simulink model "course project"  (R2023b)
settings: Solver=VariableStepAuto  StartTime=0.0  StopTime=2  RelTol=1e-3
libraries: simulink x1
(part 2 of 2)

== system course project/Register12/JCK-Trigger2 ==
  Set J : Inport
  Control C : Inport  Port=2
  Reset K : Inport  Port=3
  Logical Operator1 : Logic  Operator=NAND  Inputs=3  AllPortsSameDT=off  OutDataTypeStr=boolean
  Logical Operator2 : Logic  Operator=NAND  AllPortsSameDT=off  OutDataTypeStr=boolean
  Logical Operator3 : Logic  Operator=NAND  AllPortsSameDT=off  OutDataTypeStr=boolean
  Logical Operator5 : Logic  Operator=NAND  Inputs=3  AllPortsSameDT=off  OutDataTypeStr=boolean
  Memory : Memory
  Non-Inverted : Outport
  wires:
  Memory/1 -> Logical Operator5/2, Logical Operator3/1  "Feedback"
  Logical Operator1/1 -> Logical Operator2/1  "R"
  Logical Operator2/1 -> Non-Inverted/1, Memory/1
  Logical Operator3/1 -> Logical Operator1/2, Logical Operator2/2  "Feedback"
  Logical Operator5/1 -> Logical Operator3/2
  Set J/1 -> Logical Operator1/1
  Reset K/1 -> Logical Operator5/1
  Control C/1 -> Logical Operator5/3, Logical Operator1/3

== system course project/Register12/JCK-Trigger3 ==
  Set J : Inport
  Control C : Inport  Port=2
  Reset K : Inport  Port=3
  Logical Operator1 : Logic  Operator=NAND  Inputs=3  AllPortsSameDT=off  OutDataTypeStr=boolean
  Logical Operator2 : Logic  Operator=NAND  AllPortsSameDT=off  OutDataTypeStr=boolean
  Logical Operator3 : Logic  Operator=NAND  AllPortsSameDT=off  OutDataTypeStr=boolean
  Logical Operator5 : Logic  Operator=NAND  Inputs=3  AllPortsSameDT=off  OutDataTypeStr=boolean
  Memory : Memory
  Non-Inverted : Outport
  wires:
  Memory/1 -> Logical Operator5/2, Logical Operator3/1  "Feedback"
  Logical Operator1/1 -> Logical Operator2/1  "R"
  Logical Operator2/1 -> Non-Inverted/1, Memory/1
  Logical Operator3/1 -> Logical Operator1/2, Logical Operator2/2  "Feedback"
  Logical Operator5/1 -> Logical Operator3/2
  Set J/1 -> Logical Operator1/1
  Reset K/1 -> Logical Operator5/1
  Control C/1 -> Logical Operator5/3, Logical Operator1/3

== system course project/Register13/JCK-Trigger ==
  Set J : Inport
  Control C : Inport  Port=2
  Reset K : Inport  Port=3
  Logical Operator1 : Logic  Operator=NAND  Inputs=3  AllPortsSameDT=off  OutDataTypeStr=boolean
  Logical Operator2 : Logic  Operator=NAND  AllPortsSameDT=off  OutDataTypeStr=boolean
  Logical Operator3 : Logic  Operator=NAND  AllPortsSameDT=off  OutDataTypeStr=boolean
  Logical Operator5 : Logic  Operator=NAND  Inputs=3  AllPortsSameDT=off  OutDataTypeStr=boolean
  Memory : Memory
  Non-Inverted : Outport
  wires:
  Memory/1 -> Logical Operator5/2, Logical Operator3/1  "Feedback"
  Logical Operator1/1 -> Logical Operator2/1  "R"
  Logical Operator2/1 -> Non-Inverted/1, Memory/1
  Logical Operator3/1 -> Logical Operator1/2, Logical Operator2/2  "Feedback"
  Logical Operator5/1 -> Logical Operator3/2
  Set J/1 -> Logical Operator1/1
  Reset K/1 -> Logical Operator5/1
  Control C/1 -> Logical Operator5/3, Logical Operator1/3

== system course project/Register13/JCK-Trigger1 ==
  Set J : Inport
  Control C : Inport  Port=2
  Reset K : Inport  Port=3
  Logical Operator1 : Logic  Operator=NAND  Inputs=3  AllPortsSameDT=off  OutDataTypeStr=boolean
  Logical Operator2 : Logic  Operator=NAND  AllPortsSameDT=off  OutDataTypeStr=boolean
  Logical Operator3 : Logic  Operator=NAND  AllPortsSameDT=off  OutDataTypeStr=boolean
  Logical Operator5 : Logic  Operator=NAND  Inputs=3  AllPortsSameDT=off  OutDataTypeStr=boolean
  Memory : Memory
  Non-Inverted : Outport
  wires:
  Memory/1 -> Logical Operator5/2, Logical Operator3/1  "Feedback"
  Logical Operator1/1 -> Logical Operator2/1  "R"
  Logical Operator2/1 -> Non-Inverted/1, Memory/1
  Logical Operator3/1 -> Logical Operator1/2, Logical Operator2/2  "Feedback"
  Logical Operator5/1 -> Logical Operator3/2
  Set J/1 -> Logical Operator1/1
  Reset K/1 -> Logical Operator5/1
  Control C/1 -> Logical Operator5/3, Logical Operator1/3

== system course project/Register13/JCK-Trigger2 ==
  Set J : Inport
  Control C : Inport  Port=2
  Reset K : Inport  Port=3
  Logical Operator1 : Logic  Operator=NAND  Inputs=3  AllPortsSameDT=off  OutDataTypeStr=boolean
  Logical Operator2 : Logic  Operator=NAND  AllPortsSameDT=off  OutDataTypeStr=boolean
  Logical Operator3 : Logic  Operator=NAND  AllPortsSameDT=off  OutDataTypeStr=boolean
  Logical Operator5 : Logic  Operator=NAND  Inputs=3  AllPortsSameDT=off  OutDataTypeStr=boolean
  Memory : Memory
  Non-Inverted : Outport
  wires:
  Memory/1 -> Logical Operator5/2, Logical Operator3/1  "Feedback"
  Logical Operator1/1 -> Logical Operator2/1  "R"
  Logical Operator2/1 -> Non-Inverted/1, Memory/1
  Logical Operator3/1 -> Logical Operator1/2, Logical Operator2/2  "Feedback"
  Logical Operator5/1 -> Logical Operator3/2
  Set J/1 -> Logical Operator1/1
  Reset K/1 -> Logical Operator5/1
  Control C/1 -> Logical Operator5/3, Logical Operator1/3

== system course project/Register13/JCK-Trigger3 ==
  Set J : Inport
  Control C : Inport  Port=2
  Reset K : Inport  Port=3
  Logical Operator1 : Logic  Operator=NAND  Inputs=3  AllPortsSameDT=off  OutDataTypeStr=boolean
  Logical Operator2 : Logic  Operator=NAND  AllPortsSameDT=off  OutDataTypeStr=boolean
  Logical Operator3 : Logic  Operator=NAND  AllPortsSameDT=off  OutDataTypeStr=boolean
  Logical Operator5 : Logic  Operator=NAND  Inputs=3  AllPortsSameDT=off  OutDataTypeStr=boolean
  Memory : Memory
  Non-Inverted : Outport
  wires:
  Memory/1 -> Logical Operator5/2, Logical Operator3/1  "Feedback"
  Logical Operator1/1 -> Logical Operator2/1  "R"
  Logical Operator2/1 -> Non-Inverted/1, Memory/1
  Logical Operator3/1 -> Logical Operator1/2, Logical Operator2/2  "Feedback"
  Logical Operator5/1 -> Logical Operator3/2
  Set J/1 -> Logical Operator1/1
  Reset K/1 -> Logical Operator5/1
  Control C/1 -> Logical Operator5/3, Logical Operator1/3

== system course project/Register14/JCK-Trigger ==
  Set J : Inport
  Control C : Inport  Port=2
  Reset K : Inport  Port=3
  Logical Operator1 : Logic  Operator=NAND  Inputs=3  AllPortsSameDT=off  OutDataTypeStr=boolean
  Logical Operator2 : Logic  Operator=NAND  AllPortsSameDT=off  OutDataTypeStr=boolean
  Logical Operator3 : Logic  Operator=NAND  AllPortsSameDT=off  OutDataTypeStr=boolean
  Logical Operator5 : Logic  Operator=NAND  Inputs=3  AllPortsSameDT=off  OutDataTypeStr=boolean
  Memory : Memory
  Non-Inverted : Outport
  wires:
  Memory/1 -> Logical Operator5/2, Logical Operator3/1  "Feedback"
  Logical Operator1/1 -> Logical Operator2/1  "R"
  Logical Operator2/1 -> Non-Inverted/1, Memory/1
  Logical Operator3/1 -> Logical Operator1/2, Logical Operator2/2  "Feedback"
  Logical Operator5/1 -> Logical Operator3/2
  Set J/1 -> Logical Operator1/1
  Reset K/1 -> Logical Operator5/1
  Control C/1 -> Logical Operator5/3, Logical Operator1/3

== system course project/Register14/JCK-Trigger1 ==
  Set J : Inport
  Control C : Inport  Port=2
  Reset K : Inport  Port=3
  Logical Operator1 : Logic  Operator=NAND  Inputs=3  AllPortsSameDT=off  OutDataTypeStr=boolean
  Logical Operator2 : Logic  Operator=NAND  AllPortsSameDT=off  OutDataTypeStr=boolean
  Logical Operator3 : Logic  Operator=NAND  AllPortsSameDT=off  OutDataTypeStr=boolean
  Logical Operator5 : Logic  Operator=NAND  Inputs=3  AllPortsSameDT=off  OutDataTypeStr=boolean
  Memory : Memory
  Non-Inverted : Outport
  wires:
  Memory/1 -> Logical Operator5/2, Logical Operator3/1  "Feedback"
  Logical Operator1/1 -> Logical Operator2/1  "R"
  Logical Operator2/1 -> Non-Inverted/1, Memory/1
  Logical Operator3/1 -> Logical Operator1/2, Logical Operator2/2  "Feedback"
  Logical Operator5/1 -> Logical Operator3/2
  Set J/1 -> Logical Operator1/1
  Reset K/1 -> Logical Operator5/1
  Control C/1 -> Logical Operator5/3, Logical Operator1/3

== system course project/Register14/JCK-Trigger2 ==
  Set J : Inport
  Control C : Inport  Port=2
  Reset K : Inport  Port=3
  Logical Operator1 : Logic  Operator=NAND  Inputs=3  AllPortsSameDT=off  OutDataTypeStr=boolean
  Logical Operator2 : Logic  Operator=NAND  AllPortsSameDT=off  OutDataTypeStr=boolean
  Logical Operator3 : Logic  Operator=NAND  AllPortsSameDT=off  OutDataTypeStr=boolean
  Logical Operator5 : Logic  Operator=NAND  Inputs=3  AllPortsSameDT=off  OutDataTypeStr=boolean
  Memory : Memory
  Non-Inverted : Outport
  wires:
  Memory/1 -> Logical Operator5/2, Logical Operator3/1  "Feedback"
  Logical Operator1/1 -> Logical Operator2/1  "R"
  Logical Operator2/1 -> Non-Inverted/1, Memory/1
  Logical Operator3/1 -> Logical Operator1/2, Logical Operator2/2  "Feedback"
  Logical Operator5/1 -> Logical Operator3/2
  Set J/1 -> Logical Operator1/1
  Reset K/1 -> Logical Operator5/1
  Control C/1 -> Logical Operator5/3, Logical Operator1/3

== system course project/Register14/JCK-Trigger3 ==
  Set J : Inport
  Control C : Inport  Port=2
  Reset K : Inport  Port=3
  Logical Operator1 : Logic  Operator=NAND  Inputs=3  AllPortsSameDT=off  OutDataTypeStr=boolean
  Logical Operator2 : Logic  Operator=NAND  AllPortsSameDT=off  OutDataTypeStr=boolean
  Logical Operator3 : Logic  Operator=NAND  AllPortsSameDT=off  OutDataTypeStr=boolean
  Logical Operator5 : Logic  Operator=NAND  Inputs=3  AllPortsSameDT=off  OutDataTypeStr=boolean
  Memory : Memory
  Non-Inverted : Outport
  wires:
  Memory/1 -> Logical Operator5/2, Logical Operator3/1  "Feedback"
  Logical Operator1/1 -> Logical Operator2/1  "R"
  Logical Operator2/1 -> Non-Inverted/1, Memory/1
  Logical Operator3/1 -> Logical Operator1/2, Logical Operator2/2  "Feedback"
  Logical Operator5/1 -> Logical Operator3/2
  Set J/1 -> Logical Operator1/1
  Reset K/1 -> Logical Operator5/1
  Control C/1 -> Logical Operator5/3, Logical Operator1/3

== system course project/Register15/JCK-Trigger ==
  Set J : Inport
  Control C : Inport  Port=2
  Reset K : Inport  Port=3
  Logical Operator1 : Logic  Operator=NAND  Inputs=3  AllPortsSameDT=off  OutDataTypeStr=boolean
  Logical Operator2 : Logic  Operator=NAND  AllPortsSameDT=off  OutDataTypeStr=boolean
  Logical Operator3 : Logic  Operator=NAND  AllPortsSameDT=off  OutDataTypeStr=boolean
  Logical Operator5 : Logic  Operator=NAND  Inputs=3  AllPortsSameDT=off  OutDataTypeStr=boolean
  Memory : Memory
  Non-Inverted : Outport
  wires:
  Memory/1 -> Logical Operator5/2, Logical Operator3/1  "Feedback"
  Logical Operator1/1 -> Logical Operator2/1  "R"
  Logical Operator2/1 -> Non-Inverted/1, Memory/1
  Logical Operator3/1 -> Logical Operator1/2, Logical Operator2/2  "Feedback"
  Logical Operator5/1 -> Logical Operator3/2
  Set J/1 -> Logical Operator1/1
  Reset K/1 -> Logical Operator5/1
  Control C/1 -> Logical Operator5/3, Logical Operator1/3

== system course project/Register15/JCK-Trigger1 ==
  Set J : Inport
  Control C : Inport  Port=2
  Reset K : Inport  Port=3
  Logical Operator1 : Logic  Operator=NAND  Inputs=3  AllPortsSameDT=off  OutDataTypeStr=boolean
  Logical Operator2 : Logic  Operator=NAND  AllPortsSameDT=off  OutDataTypeStr=boolean
  Logical Operator3 : Logic  Operator=NAND  AllPortsSameDT=off  OutDataTypeStr=boolean
  Logical Operator5 : Logic  Operator=NAND  Inputs=3  AllPortsSameDT=off  OutDataTypeStr=boolean
  Memory : Memory
  Non-Inverted : Outport
  wires:
  Memory/1 -> Logical Operator5/2, Logical Operator3/1  "Feedback"
  Logical Operator1/1 -> Logical Operator2/1  "R"
  Logical Operator2/1 -> Non-Inverted/1, Memory/1
  Logical Operator3/1 -> Logical Operator1/2, Logical Operator2/2  "Feedback"
  Logical Operator5/1 -> Logical Operator3/2
  Set J/1 -> Logical Operator1/1
  Reset K/1 -> Logical Operator5/1
  Control C/1 -> Logical Operator5/3, Logical Operator1/3

== system course project/Register15/JCK-Trigger2 ==
  Set J : Inport
  Control C : Inport  Port=2
  Reset K : Inport  Port=3
  Logical Operator1 : Logic  Operator=NAND  Inputs=3  AllPortsSameDT=off  OutDataTypeStr=boolean
  Logical Operator2 : Logic  Operator=NAND  AllPortsSameDT=off  OutDataTypeStr=boolean
  Logical Operator3 : Logic  Operator=NAND  AllPortsSameDT=off  OutDataTypeStr=boolean
  Logical Operator5 : Logic  Operator=NAND  Inputs=3  AllPortsSameDT=off  OutDataTypeStr=boolean
  Memory : Memory
  Non-Inverted : Outport
  wires:
  Memory/1 -> Logical Operator5/2, Logical Operator3/1  "Feedback"
  Logical Operator1/1 -> Logical Operator2/1  "R"
  Logical Operator2/1 -> Non-Inverted/1, Memory/1
  Logical Operator3/1 -> Logical Operator1/2, Logical Operator2/2  "Feedback"
  Logical Operator5/1 -> Logical Operator3/2
  Set J/1 -> Logical Operator1/1
  Reset K/1 -> Logical Operator5/1
  Control C/1 -> Logical Operator5/3, Logical Operator1/3

== system course project/Register15/JCK-Trigger3 ==
  Set J : Inport
  Control C : Inport  Port=2
  Reset K : Inport  Port=3
  Logical Operator1 : Logic  Operator=NAND  Inputs=3  AllPortsSameDT=off  OutDataTypeStr=boolean
  Logical Operator2 : Logic  Operator=NAND  AllPortsSameDT=off  OutDataTypeStr=boolean
  Logical Operator3 : Logic  Operator=NAND  AllPortsSameDT=off  OutDataTypeStr=boolean
  Logical Operator5 : Logic  Operator=NAND  Inputs=3  AllPortsSameDT=off  OutDataTypeStr=boolean
  Memory : Memory
  Non-Inverted : Outport
  wires:
  Memory/1 -> Logical Operator5/2, Logical Operator3/1  "Feedback"
  Logical Operator1/1 -> Logical Operator2/1  "R"
  Logical Operator2/1 -> Non-Inverted/1, Memory/1
  Logical Operator3/1 -> Logical Operator1/2, Logical Operator2/2  "Feedback"
  Logical Operator5/1 -> Logical Operator3/2
  Set J/1 -> Logical Operator1/1
  Reset K/1 -> Logical Operator5/1
  Control C/1 -> Logical Operator5/3, Logical Operator1/3

== system course project/Register2/JCK-Trigger ==
  Set J : Inport
  Control C : Inport  Port=2
  Reset K : Inport  Port=3
  Logical Operator1 : Logic  Operator=NAND  Inputs=3  AllPortsSameDT=off  OutDataTypeStr=boolean
  Logical Operator2 : Logic  Operator=NAND  AllPortsSameDT=off  OutDataTypeStr=boolean
  Logical Operator3 : Logic  Operator=NAND  AllPortsSameDT=off  OutDataTypeStr=boolean
  Logical Operator5 : Logic  Operator=NAND  Inputs=3  AllPortsSameDT=off  OutDataTypeStr=boolean
  Memory : Memory
  Non-Inverted : Outport
  wires:
  Memory/1 -> Logical Operator5/2, Logical Operator3/1  "Feedback"
  Logical Operator1/1 -> Logical Operator2/1  "R"
  Logical Operator2/1 -> Non-Inverted/1, Memory/1
  Logical Operator3/1 -> Logical Operator1/2, Logical Operator2/2  "Feedback"
  Logical Operator5/1 -> Logical Operator3/2
  Set J/1 -> Logical Operator1/1
  Reset K/1 -> Logical Operator5/1
  Control C/1 -> Logical Operator5/3, Logical Operator1/3

== system course project/Register2/JCK-Trigger1 ==
  Set J : Inport
  Control C : Inport  Port=2
  Reset K : Inport  Port=3
  Logical Operator1 : Logic  Operator=NAND  Inputs=3  AllPortsSameDT=off  OutDataTypeStr=boolean
  Logical Operator2 : Logic  Operator=NAND  AllPortsSameDT=off  OutDataTypeStr=boolean
  Logical Operator3 : Logic  Operator=NAND  AllPortsSameDT=off  OutDataTypeStr=boolean
  Logical Operator5 : Logic  Operator=NAND  Inputs=3  AllPortsSameDT=off  OutDataTypeStr=boolean
  Memory : Memory
  Non-Inverted : Outport
  wires:
  Memory/1 -> Logical Operator5/2, Logical Operator3/1  "Feedback"
  Logical Operator1/1 -> Logical Operator2/1  "R"
  Logical Operator2/1 -> Non-Inverted/1, Memory/1
  Logical Operator3/1 -> Logical Operator1/2, Logical Operator2/2  "Feedback"
  Logical Operator5/1 -> Logical Operator3/2
  Set J/1 -> Logical Operator1/1
  Reset K/1 -> Logical Operator5/1
  Control C/1 -> Logical Operator5/3, Logical Operator1/3

== system course project/Register2/JCK-Trigger2 ==
  Set J : Inport
  Control C : Inport  Port=2
  Reset K : Inport  Port=3
  Logical Operator1 : Logic  Operator=NAND  Inputs=3  AllPortsSameDT=off  OutDataTypeStr=boolean
  Logical Operator2 : Logic  Operator=NAND  AllPortsSameDT=off  OutDataTypeStr=boolean
  Logical Operator3 : Logic  Operator=NAND  AllPortsSameDT=off  OutDataTypeStr=boolean
  Logical Operator5 : Logic  Operator=NAND  Inputs=3  AllPortsSameDT=off  OutDataTypeStr=boolean
  Memory : Memory
  Non-Inverted : Outport
  wires:
  Memory/1 -> Logical Operator5/2, Logical Operator3/1  "Feedback"
  Logical Operator1/1 -> Logical Operator2/1  "R"
  Logical Operator2/1 -> Non-Inverted/1, Memory/1
  Logical Operator3/1 -> Logical Operator1/2, Logical Operator2/2  "Feedback"
  Logical Operator5/1 -> Logical Operator3/2
  Set J/1 -> Logical Operator1/1
  Reset K/1 -> Logical Operator5/1
  Control C/1 -> Logical Operator5/3, Logical Operator1/3

== system course project/Register2/JCK-Trigger3 ==
  Set J : Inport
  Control C : Inport  Port=2
  Reset K : Inport  Port=3
  Logical Operator1 : Logic  Operator=NAND  Inputs=3  AllPortsSameDT=off  OutDataTypeStr=boolean
  Logical Operator2 : Logic  Operator=NAND  AllPortsSameDT=off  OutDataTypeStr=boolean
  Logical Operator3 : Logic  Operator=NAND  AllPortsSameDT=off  OutDataTypeStr=boolean
  Logical Operator5 : Logic  Operator=NAND  Inputs=3  AllPortsSameDT=off  OutDataTypeStr=boolean
  Memory : Memory
  Non-Inverted : Outport
  wires:
  Memory/1 -> Logical Operator5/2, Logical Operator3/1  "Feedback"
  Logical Operator1/1 -> Logical Operator2/1  "R"
  Logical Operator2/1 -> Non-Inverted/1, Memory/1
  Logical Operator3/1 -> Logical Operator1/2, Logical Operator2/2  "Feedback"
  Logical Operator5/1 -> Logical Operator3/2
  Set J/1 -> Logical Operator1/1
  Reset K/1 -> Logical Operator5/1
  Control C/1 -> Logical Operator5/3, Logical Operator1/3

== system course project/Register3/JCK-Trigger ==
  Set J : Inport
  Control C : Inport  Port=2
  Reset K : Inport  Port=3
  Logical Operator1 : Logic  Operator=NAND  Inputs=3  AllPortsSameDT=off  OutDataTypeStr=boolean
  Logical Operator2 : Logic  Operator=NAND  AllPortsSameDT=off  OutDataTypeStr=boolean
  Logical Operator3 : Logic  Operator=NAND  AllPortsSameDT=off  OutDataTypeStr=boolean
  Logical Operator5 : Logic  Operator=NAND  Inputs=3  AllPortsSameDT=off  OutDataTypeStr=boolean
  Memory : Memory
  Non-Inverted : Outport
  wires:
  Memory/1 -> Logical Operator5/2, Logical Operator3/1  "Feedback"
  Logical Operator1/1 -> Logical Operator2/1  "R"
  Logical Operator2/1 -> Non-Inverted/1, Memory/1
  Logical Operator3/1 -> Logical Operator1/2, Logical Operator2/2  "Feedback"
  Logical Operator5/1 -> Logical Operator3/2
  Set J/1 -> Logical Operator1/1
  Reset K/1 -> Logical Operator5/1
  Control C/1 -> Logical Operator5/3, Logical Operator1/3

== system course project/Register3/JCK-Trigger1 ==
  Set J : Inport
  Control C : Inport  Port=2
  Reset K : Inport  Port=3
  Logical Operator1 : Logic  Operator=NAND  Inputs=3  AllPortsSameDT=off  OutDataTypeStr=boolean
  Logical Operator2 : Logic  Operator=NAND  AllPortsSameDT=off  OutDataTypeStr=boolean
  Logical Operator3 : Logic  Operator=NAND  AllPortsSameDT=off  OutDataTypeStr=boolean
  Logical Operator5 : Logic  Operator=NAND  Inputs=3  AllPortsSameDT=off  OutDataTypeStr=boolean
  Memory : Memory
  Non-Inverted : Outport
  wires:
  Memory/1 -> Logical Operator5/2, Logical Operator3/1  "Feedback"
  Logical Operator1/1 -> Logical Operator2/1  "R"
  Logical Operator2/1 -> Non-Inverted/1, Memory/1
  Logical Operator3/1 -> Logical Operator1/2, Logical Operator2/2  "Feedback"
  Logical Operator5/1 -> Logical Operator3/2
  Set J/1 -> Logical Operator1/1
  Reset K/1 -> Logical Operator5/1
  Control C/1 -> Logical Operator5/3, Logical Operator1/3

== system course project/Register3/JCK-Trigger2 ==
  Set J : Inport
  Control C : Inport  Port=2
  Reset K : Inport  Port=3
  Logical Operator1 : Logic  Operator=NAND  Inputs=3  AllPortsSameDT=off  OutDataTypeStr=boolean
  Logical Operator2 : Logic  Operator=NAND  AllPortsSameDT=off  OutDataTypeStr=boolean
  Logical Operator3 : Logic  Operator=NAND  AllPortsSameDT=off  OutDataTypeStr=boolean
  Logical Operator5 : Logic  Operator=NAND  Inputs=3  AllPortsSameDT=off  OutDataTypeStr=boolean
  Memory : Memory
  Non-Inverted : Outport
  wires:
  Memory/1 -> Logical Operator5/2, Logical Operator3/1  "Feedback"
  Logical Operator1/1 -> Logical Operator2/1  "R"
  Logical Operator2/1 -> Non-Inverted/1, Memory/1
  Logical Operator3/1 -> Logical Operator1/2, Logical Operator2/2  "Feedback"
  Logical Operator5/1 -> Logical Operator3/2
  Set J/1 -> Logical Operator1/1
  Reset K/1 -> Logical Operator5/1
  Control C/1 -> Logical Operator5/3, Logical Operator1/3

== system course project/Register3/JCK-Trigger3 ==
  Set J : Inport
  Control C : Inport  Port=2
  Reset K : Inport  Port=3
  Logical Operator1 : Logic  Operator=NAND  Inputs=3  AllPortsSameDT=off  OutDataTypeStr=boolean
  Logical Operator2 : Logic  Operator=NAND  AllPortsSameDT=off  OutDataTypeStr=boolean
  Logical Operator3 : Logic  Operator=NAND  AllPortsSameDT=off  OutDataTypeStr=boolean
  Logical Operator5 : Logic  Operator=NAND  Inputs=3  AllPortsSameDT=off  OutDataTypeStr=boolean
  Memory : Memory
  Non-Inverted : Outport
  wires:
  Memory/1 -> Logical Operator5/2, Logical Operator3/1  "Feedback"
  Logical Operator1/1 -> Logical Operator2/1  "R"
  Logical Operator2/1 -> Non-Inverted/1, Memory/1
  Logical Operator3/1 -> Logical Operator1/2, Logical Operator2/2  "Feedback"
  Logical Operator5/1 -> Logical Operator3/2
  Set J/1 -> Logical Operator1/1
  Reset K/1 -> Logical Operator5/1
  Control C/1 -> Logical Operator5/3, Logical Operator1/3

== system course project/Register4/JCK-Trigger ==
  Set J : Inport
  Control C : Inport  Port=2
  Reset K : Inport  Port=3
  Logical Operator1 : Logic  Operator=NAND  Inputs=3  AllPortsSameDT=off  OutDataTypeStr=boolean
  Logical Operator2 : Logic  Operator=NAND  AllPortsSameDT=off  OutDataTypeStr=boolean
  Logical Operator3 : Logic  Operator=NAND  AllPortsSameDT=off  OutDataTypeStr=boolean
  Logical Operator5 : Logic  Operator=NAND  Inputs=3  AllPortsSameDT=off  OutDataTypeStr=boolean
  Memory : Memory
  Non-Inverted : Outport
  wires:
  Memory/1 -> Logical Operator5/2, Logical Operator3/1  "Feedback"
  Logical Operator1/1 -> Logical Operator2/1  "R"
  Logical Operator2/1 -> Non-Inverted/1, Memory/1
  Logical Operator3/1 -> Logical Operator1/2, Logical Operator2/2  "Feedback"
  Logical Operator5/1 -> Logical Operator3/2
  Set J/1 -> Logical Operator1/1
  Reset K/1 -> Logical Operator5/1
  Control C/1 -> Logical Operator5/3, Logical Operator1/3

== system course project/Register4/JCK-Trigger1 ==
  Set J : Inport
  Control C : Inport  Port=2
  Reset K : Inport  Port=3
  Logical Operator1 : Logic  Operator=NAND  Inputs=3  AllPortsSameDT=off  OutDataTypeStr=boolean
  Logical Operator2 : Logic  Operator=NAND  AllPortsSameDT=off  OutDataTypeStr=boolean
  Logical Operator3 : Logic  Operator=NAND  AllPortsSameDT=off  OutDataTypeStr=boolean
  Logical Operator5 : Logic  Operator=NAND  Inputs=3  AllPortsSameDT=off  OutDataTypeStr=boolean
  Memory : Memory
  Non-Inverted : Outport
  wires:
  Memory/1 -> Logical Operator5/2, Logical Operator3/1  "Feedback"
  Logical Operator1/1 -> Logical Operator2/1  "R"
  Logical Operator2/1 -> Non-Inverted/1, Memory/1
  Logical Operator3/1 -> Logical Operator1/2, Logical Operator2/2  "Feedback"
  Logical Operator5/1 -> Logical Operator3/2
  Set J/1 -> Logical Operator1/1
  Reset K/1 -> Logical Operator5/1
  Control C/1 -> Logical Operator5/3, Logical Operator1/3

== system course project/Register4/JCK-Trigger2 ==
  Set J : Inport
  Control C : Inport  Port=2
  Reset K : Inport  Port=3
  Logical Operator1 : Logic  Operator=NAND  Inputs=3  AllPortsSameDT=off  OutDataTypeStr=boolean
  Logical Operator2 : Logic  Operator=NAND  AllPortsSameDT=off  OutDataTypeStr=boolean
  Logical Operator3 : Logic  Operator=NAND  AllPortsSameDT=off  OutDataTypeStr=boolean
  Logical Operator5 : Logic  Operator=NAND  Inputs=3  AllPortsSameDT=off  OutDataTypeStr=boolean
  Memory : Memory
  Non-Inverted : Outport
  wires:
  Memory/1 -> Logical Operator5/2, Logical Operator3/1  "Feedback"
  Logical Operator1/1 -> Logical Operator2/1  "R"
  Logical Operator2/1 -> Non-Inverted/1, Memory/1
  Logical Operator3/1 -> Logical Operator1/2, Logical Operator2/2  "Feedback"
  Logical Operator5/1 -> Logical Operator3/2
  Set J/1 -> Logical Operator1/1
  Reset K/1 -> Logical Operator5/1
  Control C/1 -> Logical Operator5/3, Logical Operator1/3

== system course project/Register4/JCK-Trigger3 ==
  Set J : Inport
  Control C : Inport  Port=2
  Reset K : Inport  Port=3
  Logical Operator1 : Logic  Operator=NAND  Inputs=3  AllPortsSameDT=off  OutDataTypeStr=boolean
  Logical Operator2 : Logic  Operator=NAND  AllPortsSameDT=off  OutDataTypeStr=boolean
  Logical Operator3 : Logic  Operator=NAND  AllPortsSameDT=off  OutDataTypeStr=boolean
  Logical Operator5 : Logic  Operator=NAND  Inputs=3  AllPortsSameDT=off  OutDataTypeStr=boolean
  Memory : Memory
  Non-Inverted : Outport
  wires:
  Memory/1 -> Logical Operator5/2, Logical Operator3/1  "Feedback"
  Logical Operator1/1 -> Logical Operator2/1  "R"
  Logical Operator2/1 -> Non-Inverted/1, Memory/1
  Logical Operator3/1 -> Logical Operator1/2, Logical Operator2/2  "Feedback"
  Logical Operator5/1 -> Logical Operator3/2
  Set J/1 -> Logical Operator1/1
  Reset K/1 -> Logical Operator5/1
  Control C/1 -> Logical Operator5/3, Logical Operator1/3

== system course project/Register5/JCK-Trigger ==
  Set J : Inport
  Control C : Inport  Port=2
  Reset K : Inport  Port=3
  Logical Operator1 : Logic  Operator=NAND  Inputs=3  AllPortsSameDT=off  OutDataTypeStr=boolean
  Logical Operator2 : Logic  Operator=NAND  AllPortsSameDT=off  OutDataTypeStr=boolean
  Logical Operator3 : Logic  Operator=NAND  AllPortsSameDT=off  OutDataTypeStr=boolean
  Logical Operator5 : Logic  Operator=NAND  Inputs=3  AllPortsSameDT=off  OutDataTypeStr=boolean
  Memory : Memory
  Non-Inverted : Outport
  wires:
  Memory/1 -> Logical Operator5/2, Logical Operator3/1  "Feedback"
  Logical Operator1/1 -> Logical Operator2/1  "R"
  Logical Operator2/1 -> Non-Inverted/1, Memory/1
  Logical Operator3/1 -> Logical Operator1/2, Logical Operator2/2  "Feedback"
  Logical Operator5/1 -> Logical Operator3/2
  Set J/1 -> Logical Operator1/1
  Reset K/1 -> Logical Operator5/1
  Control C/1 -> Logical Operator5/3, Logical Operator1/3

== system course project/Register5/JCK-Trigger1 ==
  Set J : Inport
  Control C : Inport  Port=2
  Reset K : Inport  Port=3
  Logical Operator1 : Logic  Operator=NAND  Inputs=3  AllPortsSameDT=off  OutDataTypeStr=boolean
  Logical Operator2 : Logic  Operator=NAND  AllPortsSameDT=off  OutDataTypeStr=boolean
  Logical Operator3 : Logic  Operator=NAND  AllPortsSameDT=off  OutDataTypeStr=boolean
  Logical Operator5 : Logic  Operator=NAND  Inputs=3  AllPortsSameDT=off  OutDataTypeStr=boolean
  Memory : Memory
  Non-Inverted : Outport
  wires:
  Memory/1 -> Logical Operator5/2, Logical Operator3/1  "Feedback"
  Logical Operator1/1 -> Logical Operator2/1  "R"
  Logical Operator2/1 -> Non-Inverted/1, Memory/1
  Logical Operator3/1 -> Logical Operator1/2, Logical Operator2/2  "Feedback"
  Logical Operator5/1 -> Logical Operator3/2
  Set J/1 -> Logical Operator1/1
  Reset K/1 -> Logical Operator5/1
  Control C/1 -> Logical Operator5/3, Logical Operator1/3

== system course project/Register5/JCK-Trigger2 ==
  Set J : Inport
  Control C : Inport  Port=2
  Reset K : Inport  Port=3
  Logical Operator1 : Logic  Operator=NAND  Inputs=3  AllPortsSameDT=off  OutDataTypeStr=boolean
  Logical Operator2 : Logic  Operator=NAND  AllPortsSameDT=off  OutDataTypeStr=boolean
  Logical Operator3 : Logic  Operator=NAND  AllPortsSameDT=off  OutDataTypeStr=boolean
  Logical Operator5 : Logic  Operator=NAND  Inputs=3  AllPortsSameDT=off  OutDataTypeStr=boolean
  Memory : Memory
  Non-Inverted : Outport
  wires:
  Memory/1 -> Logical Operator5/2, Logical Operator3/1  "Feedback"
  Logical Operator1/1 -> Logical Operator2/1  "R"
  Logical Operator2/1 -> Non-Inverted/1, Memory/1
  Logical Operator3/1 -> Logical Operator1/2, Logical Operator2/2  "Feedback"
  Logical Operator5/1 -> Logical Operator3/2
  Set J/1 -> Logical Operator1/1
  Reset K/1 -> Logical Operator5/1
  Control C/1 -> Logical Operator5/3, Logical Operator1/3

== system course project/Register5/JCK-Trigger3 ==
  Set J : Inport
  Control C : Inport  Port=2
  Reset K : Inport  Port=3
  Logical Operator1 : Logic  Operator=NAND  Inputs=3  AllPortsSameDT=off  OutDataTypeStr=boolean
  Logical Operator2 : Logic  Operator=NAND  AllPortsSameDT=off  OutDataTypeStr=boolean
  Logical Operator3 : Logic  Operator=NAND  AllPortsSameDT=off  OutDataTypeStr=boolean
  Logical Operator5 : Logic  Operator=NAND  Inputs=3  AllPortsSameDT=off  OutDataTypeStr=boolean
  Memory : Memory
  Non-Inverted : Outport
  wires:
  Memory/1 -> Logical Operator5/2, Logical Operator3/1  "Feedback"
  Logical Operator1/1 -> Logical Operator2/1  "R"
  Logical Operator2/1 -> Non-Inverted/1, Memory/1
  Logical Operator3/1 -> Logical Operator1/2, Logical Operator2/2  "Feedback"
  Logical Operator5/1 -> Logical Operator3/2
  Set J/1 -> Logical Operator1/1
  Reset K/1 -> Logical Operator5/1
  Control C/1 -> Logical Operator5/3, Logical Operator1/3

== system course project/Register6/JCK-Trigger ==
  Set J : Inport
  Control C : Inport  Port=2
  Reset K : Inport  Port=3
  Logical Operator1 : Logic  Operator=NAND  Inputs=3  AllPortsSameDT=off  OutDataTypeStr=boolean
  Logical Operator2 : Logic  Operator=NAND  AllPortsSameDT=off  OutDataTypeStr=boolean
  Logical Operator3 : Logic  Operator=NAND  AllPortsSameDT=off  OutDataTypeStr=boolean
  Logical Operator5 : Logic  Operator=NAND  Inputs=3  AllPortsSameDT=off  OutDataTypeStr=boolean
  Memory : Memory
  Non-Inverted : Outport
  wires:
  Memory/1 -> Logical Operator5/2, Logical Operator3/1  "Feedback"
  Logical Operator1/1 -> Logical Operator2/1  "R"
  Logical Operator2/1 -> Non-Inverted/1, Memory/1
  Logical Operator3/1 -> Logical Operator1/2, Logical Operator2/2  "Feedback"
  Logical Operator5/1 -> Logical Operator3/2
  Set J/1 -> Logical Operator1/1
  Reset K/1 -> Logical Operator5/1
  Control C/1 -> Logical Operator5/3, Logical Operator1/3

== system course project/Register6/JCK-Trigger1 ==
  Set J : Inport
  Control C : Inport  Port=2
  Reset K : Inport  Port=3
  Logical Operator1 : Logic  Operator=NAND  Inputs=3  AllPortsSameDT=off  OutDataTypeStr=boolean
  Logical Operator2 : Logic  Operator=NAND  AllPortsSameDT=off  OutDataTypeStr=boolean
  Logical Operator3 : Logic  Operator=NAND  AllPortsSameDT=off  OutDataTypeStr=boolean
  Logical Operator5 : Logic  Operator=NAND  Inputs=3  AllPortsSameDT=off  OutDataTypeStr=boolean
  Memory : Memory
  Non-Inverted : Outport
  wires:
  Memory/1 -> Logical Operator5/2, Logical Operator3/1  "Feedback"
  Logical Operator1/1 -> Logical Operator2/1  "R"
  Logical Operator2/1 -> Non-Inverted/1, Memory/1
  Logical Operator3/1 -> Logical Operator1/2, Logical Operator2/2  "Feedback"
  Logical Operator5/1 -> Logical Operator3/2
  Set J/1 -> Logical Operator1/1
  Reset K/1 -> Logical Operator5/1
  Control C/1 -> Logical Operator5/3, Logical Operator1/3

== system course project/Register6/JCK-Trigger2 ==
  Set J : Inport
  Control C : Inport  Port=2
  Reset K : Inport  Port=3
  Logical Operator1 : Logic  Operator=NAND  Inputs=3  AllPortsSameDT=off  OutDataTypeStr=boolean
  Logical Operator2 : Logic  Operator=NAND  AllPortsSameDT=off  OutDataTypeStr=boolean
  Logical Operator3 : Logic  Operator=NAND  AllPortsSameDT=off  OutDataTypeStr=boolean
  Logical Operator5 : Logic  Operator=NAND  Inputs=3  AllPortsSameDT=off  OutDataTypeStr=boolean
  Memory : Memory
  Non-Inverted : Outport
  wires:
  Memory/1 -> Logical Operator5/2, Logical Operator3/1  "Feedback"
  Logical Operator1/1 -> Logical Operator2/1  "R"
  Logical Operator2/1 -> Non-Inverted/1, Memory/1
  Logical Operator3/1 -> Logical Operator1/2, Logical Operator2/2  "Feedback"
  Logical Operator5/1 -> Logical Operator3/2
  Set J/1 -> Logical Operator1/1
  Reset K/1 -> Logical Operator5/1
  Control C/1 -> Logical Operator5/3, Logical Operator1/3

== system course project/Register6/JCK-Trigger3 ==
  Set J : Inport
  Control C : Inport  Port=2
  Reset K : Inport  Port=3
  Logical Operator1 : Logic  Operator=NAND  Inputs=3  AllPortsSameDT=off  OutDataTypeStr=boolean
  Logical Operator2 : Logic  Operator=NAND  AllPortsSameDT=off  OutDataTypeStr=boolean
  Logical Operator3 : Logic  Operator=NAND  AllPortsSameDT=off  OutDataTypeStr=boolean
  Logical Operator5 : Logic  Operator=NAND  Inputs=3  AllPortsSameDT=off  OutDataTypeStr=boolean
  Memory : Memory
  Non-Inverted : Outport
  wires:
  Memory/1 -> Logical Operator5/2, Logical Operator3/1  "Feedback"
  Logical Operator1/1 -> Logical Operator2/1  "R"
  Logical Operator2/1 -> Non-Inverted/1, Memory/1
  Logical Operator3/1 -> Logical Operator1/2, Logical Operator2/2  "Feedback"
  Logical Operator5/1 -> Logical Operator3/2
  Set J/1 -> Logical Operator1/1
  Reset K/1 -> Logical Operator5/1
  Control C/1 -> Logical Operator5/3, Logical Operator1/3

== system course project/Register7/JCK-Trigger ==
  Set J : Inport
  Control C : Inport  Port=2
  Reset K : Inport  Port=3
  Logical Operator1 : Logic  Operator=NAND  Inputs=3  AllPortsSameDT=off  OutDataTypeStr=boolean
  Logical Operator2 : Logic  Operator=NAND  AllPortsSameDT=off  OutDataTypeStr=boolean
  Logical Operator3 : Logic  Operator=NAND  AllPortsSameDT=off  OutDataTypeStr=boolean
  Logical Operator5 : Logic  Operator=NAND  Inputs=3  AllPortsSameDT=off  OutDataTypeStr=boolean
  Memory : Memory
  Non-Inverted : Outport
  wires:
  Memory/1 -> Logical Operator5/2, Logical Operator3/1  "Feedback"
  Logical Operator1/1 -> Logical Operator2/1  "R"
  Logical Operator2/1 -> Non-Inverted/1, Memory/1
  Logical Operator3/1 -> Logical Operator1/2, Logical Operator2/2  "Feedback"
  Logical Operator5/1 -> Logical Operator3/2
  Set J/1 -> Logical Operator1/1
  Reset K/1 -> Logical Operator5/1
  Control C/1 -> Logical Operator5/3, Logical Operator1/3

== system course project/Register7/JCK-Trigger1 ==
  Set J : Inport
  Control C : Inport  Port=2
  Reset K : Inport  Port=3
  Logical Operator1 : Logic  Operator=NAND  Inputs=3  AllPortsSameDT=off  OutDataTypeStr=boolean
  Logical Operator2 : Logic  Operator=NAND  AllPortsSameDT=off  OutDataTypeStr=boolean
  Logical Operator3 : Logic  Operator=NAND  AllPortsSameDT=off  OutDataTypeStr=boolean
  Logical Operator5 : Logic  Operator=NAND  Inputs=3  AllPortsSameDT=off  OutDataTypeStr=boolean
  Memory : Memory
  Non-Inverted : Outport
  wires:
  Memory/1 -> Logical Operator5/2, Logical Operator3/1  "Feedback"
  Logical Operator1/1 -> Logical Operator2/1  "R"
  Logical Operator2/1 -> Non-Inverted/1, Memory/1
  Logical Operator3/1 -> Logical Operator1/2, Logical Operator2/2  "Feedback"
  Logical Operator5/1 -> Logical Operator3/2
  Set J/1 -> Logical Operator1/1
  Reset K/1 -> Logical Operator5/1
  Control C/1 -> Logical Operator5/3, Logical Operator1/3

== system course project/Register7/JCK-Trigger2 ==
  Set J : Inport
  Control C : Inport  Port=2
  Reset K : Inport  Port=3
  Logical Operator1 : Logic  Operator=NAND  Inputs=3  AllPortsSameDT=off  OutDataTypeStr=boolean
  Logical Operator2 : Logic  Operator=NAND  AllPortsSameDT=off  OutDataTypeStr=boolean
  Logical Operator3 : Logic  Operator=NAND  AllPortsSameDT=off  OutDataTypeStr=boolean
  Logical Operator5 : Logic  Operator=NAND  Inputs=3  AllPortsSameDT=off  OutDataTypeStr=boolean
  Memory : Memory
  Non-Inverted : Outport
  wires:
  Memory/1 -> Logical Operator5/2, Logical Operator3/1  "Feedback"
  Logical Operator1/1 -> Logical Operator2/1  "R"
  Logical Operator2/1 -> Non-Inverted/1, Memory/1
  Logical Operator3/1 -> Logical Operator1/2, Logical Operator2/2  "Feedback"
  Logical Operator5/1 -> Logical Operator3/2
  Set J/1 -> Logical Operator1/1
  Reset K/1 -> Logical Operator5/1
  Control C/1 -> Logical Operator5/3, Logical Operator1/3

== system course project/Register7/JCK-Trigger3 ==
  Set J : Inport
  Control C : Inport  Port=2
  Reset K : Inport  Port=3
  Logical Operator1 : Logic  Operator=NAND  Inputs=3  AllPortsSameDT=off  OutDataTypeStr=boolean
  Logical Operator2 : Logic  Operator=NAND  AllPortsSameDT=off  OutDataTypeStr=boolean
  Logical Operator3 : Logic  Operator=NAND  AllPortsSameDT=off  OutDataTypeStr=boolean
  Logical Operator5 : Logic  Operator=NAND  Inputs=3  AllPortsSameDT=off  OutDataTypeStr=boolean
  Memory : Memory
  Non-Inverted : Outport
  wires:
  Memory/1 -> Logical Operator5/2, Logical Operator3/1  "Feedback"
  Logical Operator1/1 -> Logical Operator2/1  "R"
  Logical Operator2/1 -> Non-Inverted/1, Memory/1
  Logical Operator3/1 -> Logical Operator1/2, Logical Operator2/2  "Feedback"
  Logical Operator5/1 -> Logical Operator3/2
  Set J/1 -> Logical Operator1/1
  Reset K/1 -> Logical Operator5/1
  Control C/1 -> Logical Operator5/3, Logical Operator1/3

== system course project/Register8/JCK-Trigger ==
  Set J : Inport
  Control C : Inport  Port=2
  Reset K : Inport  Port=3
  Logical Operator1 : Logic  Operator=NAND  Inputs=3  AllPortsSameDT=off  OutDataTypeStr=boolean
  Logical Operator2 : Logic  Operator=NAND  AllPortsSameDT=off  OutDataTypeStr=boolean
  Logical Operator3 : Logic  Operator=NAND  AllPortsSameDT=off  OutDataTypeStr=boolean
  Logical Operator5 : Logic  Operator=NAND  Inputs=3  AllPortsSameDT=off  OutDataTypeStr=boolean
  Memory : Memory
  Non-Inverted : Outport
  wires:
  Memory/1 -> Logical Operator5/2, Logical Operator3/1  "Feedback"
  Logical Operator1/1 -> Logical Operator2/1  "R"
  Logical Operator2/1 -> Non-Inverted/1, Memory/1
  Logical Operator3/1 -> Logical Operator1/2, Logical Operator2/2  "Feedback"
  Logical Operator5/1 -> Logical Operator3/2
  Set J/1 -> Logical Operator1/1
  Reset K/1 -> Logical Operator5/1
  Control C/1 -> Logical Operator5/3, Logical Operator1/3

== system course project/Register8/JCK-Trigger1 ==
  Set J : Inport
  Control C : Inport  Port=2
  Reset K : Inport  Port=3
  Logical Operator1 : Logic  Operator=NAND  Inputs=3  AllPortsSameDT=off  OutDataTypeStr=boolean
  Logical Operator2 : Logic  Operator=NAND  AllPortsSameDT=off  OutDataTypeStr=boolean
  Logical Operator3 : Logic  Operator=NAND  AllPortsSameDT=off  OutDataTypeStr=boolean
  Logical Operator5 : Logic  Operator=NAND  Inputs=3  AllPortsSameDT=off  OutDataTypeStr=boolean
  Memory : Memory
  Non-Inverted : Outport
  wires:
  Memory/1 -> Logical Operator5/2, Logical Operator3/1  "Feedback"
  Logical Operator1/1 -> Logical Operator2/1  "R"
  Logical Operator2/1 -> Non-Inverted/1, Memory/1
  Logical Operator3/1 -> Logical Operator1/2, Logical Operator2/2  "Feedback"
  Logical Operator5/1 -> Logical Operator3/2
  Set J/1 -> Logical Operator1/1
  Reset K/1 -> Logical Operator5/1
  Control C/1 -> Logical Operator5/3, Logical Operator1/3

== system course project/Register8/JCK-Trigger2 ==
  Set J : Inport
  Control C : Inport  Port=2
  Reset K : Inport  Port=3
  Logical Operator1 : Logic  Operator=NAND  Inputs=3  AllPortsSameDT=off  OutDataTypeStr=boolean
  Logical Operator2 : Logic  Operator=NAND  AllPortsSameDT=off  OutDataTypeStr=boolean
  Logical Operator3 : Logic  Operator=NAND  AllPortsSameDT=off  OutDataTypeStr=boolean
  Logical Operator5 : Logic  Operator=NAND  Inputs=3  AllPortsSameDT=off  OutDataTypeStr=boolean
  Memory : Memory
  Non-Inverted : Outport
  wires:
  Memory/1 -> Logical Operator5/2, Logical Operator3/1  "Feedback"
  Logical Operator1/1 -> Logical Operator2/1  "R"
  Logical Operator2/1 -> Non-Inverted/1, Memory/1
  Logical Operator3/1 -> Logical Operator1/2, Logical Operator2/2  "Feedback"
  Logical Operator5/1 -> Logical Operator3/2
  Set J/1 -> Logical Operator1/1
  Reset K/1 -> Logical Operator5/1
  Control C/1 -> Logical Operator5/3, Logical Operator1/3

== system course project/Register8/JCK-Trigger3 ==
  Set J : Inport
  Control C : Inport  Port=2
  Reset K : Inport  Port=3
  Logical Operator1 : Logic  Operator=NAND  Inputs=3  AllPortsSameDT=off  OutDataTypeStr=boolean
  Logical Operator2 : Logic  Operator=NAND  AllPortsSameDT=off  OutDataTypeStr=boolean
  Logical Operator3 : Logic  Operator=NAND  AllPortsSameDT=off  OutDataTypeStr=boolean
  Logical Operator5 : Logic  Operator=NAND  Inputs=3  AllPortsSameDT=off  OutDataTypeStr=boolean
  Memory : Memory
  Non-Inverted : Outport
  wires:
  Memory/1 -> Logical Operator5/2, Logical Operator3/1  "Feedback"
  Logical Operator1/1 -> Logical Operator2/1  "R"
  Logical Operator2/1 -> Non-Inverted/1, Memory/1
  Logical Operator3/1 -> Logical Operator1/2, Logical Operator2/2  "Feedback"
  Logical Operator5/1 -> Logical Operator3/2
  Set J/1 -> Logical Operator1/1
  Reset K/1 -> Logical Operator5/1
  Control C/1 -> Logical Operator5/3, Logical Operator1/3

== system course project/Register9/JCK-Trigger ==
  Set J : Inport
  Control C : Inport  Port=2
  Reset K : Inport  Port=3
  Logical Operator1 : Logic  Operator=NAND  Inputs=3  AllPortsSameDT=off  OutDataTypeStr=boolean
  Logical Operator2 : Logic  Operator=NAND  AllPortsSameDT=off  OutDataTypeStr=boolean
  Logical Operator3 : Logic  Operator=NAND  AllPortsSameDT=off  OutDataTypeStr=boolean
  Logical Operator5 : Logic  Operator=NAND  Inputs=3  AllPortsSameDT=off  OutDataTypeStr=boolean
  Memory : Memory
  Non-Inverted : Outport
  wires:
  Memory/1 -> Logical Operator5/2, Logical Operator3/1  "Feedback"
  Logical Operator1/1 -> Logical Operator2/1  "R"
  Logical Operator2/1 -> Non-Inverted/1, Memory/1
  Logical Operator3/1 -> Logical Operator1/2, Logical Operator2/2  "Feedback"
  Logical Operator5/1 -> Logical Operator3/2
  Set J/1 -> Logical Operator1/1
  Reset K/1 -> Logical Operator5/1
  Control C/1 -> Logical Operator5/3, Logical Operator1/3

== system course project/Register9/JCK-Trigger1 ==
  Set J : Inport
  Control C : Inport  Port=2
  Reset K : Inport  Port=3
  Logical Operator1 : Logic  Operator=NAND  Inputs=3  AllPortsSameDT=off  OutDataTypeStr=boolean
  Logical Operator2 : Logic  Operator=NAND  AllPortsSameDT=off  OutDataTypeStr=boolean
  Logical Operator3 : Logic  Operator=NAND  AllPortsSameDT=off  OutDataTypeStr=boolean
  Logical Operator5 : Logic  Operator=NAND  Inputs=3  AllPortsSameDT=off  OutDataTypeStr=boolean
  Memory : Memory
  Non-Inverted : Outport
  wires:
  Memory/1 -> Logical Operator5/2, Logical Operator3/1  "Feedback"
  Logical Operator1/1 -> Logical Operator2/1  "R"
  Logical Operator2/1 -> Non-Inverted/1, Memory/1
  Logical Operator3/1 -> Logical Operator1/2, Logical Operator2/2  "Feedback"
  Logical Operator5/1 -> Logical Operator3/2
  Set J/1 -> Logical Operator1/1
  Reset K/1 -> Logical Operator5/1
  Control C/1 -> Logical Operator5/3, Logical Operator1/3

== system course project/Register9/JCK-Trigger2 ==
  Set J : Inport
  Control C : Inport  Port=2
  Reset K : Inport  Port=3
  Logical Operator1 : Logic  Operator=NAND  Inputs=3  AllPortsSameDT=off  OutDataTypeStr=boolean
  Logical Operator2 : Logic  Operator=NAND  AllPortsSameDT=off  OutDataTypeStr=boolean
  Logical Operator3 : Logic  Operator=NAND  AllPortsSameDT=off  OutDataTypeStr=boolean
  Logical Operator5 : Logic  Operator=NAND  Inputs=3  AllPortsSameDT=off  OutDataTypeStr=boolean
  Memory : Memory
  Non-Inverted : Outport
  wires:
  Memory/1 -> Logical Operator5/2, Logical Operator3/1  "Feedback"
  Logical Operator1/1 -> Logical Operator2/1  "R"
  Logical Operator2/1 -> Non-Inverted/1, Memory/1
  Logical Operator3/1 -> Logical Operator1/2, Logical Operator2/2  "Feedback"
  Logical Operator5/1 -> Logical Operator3/2
  Set J/1 -> Logical Operator1/1
  Reset K/1 -> Logical Operator5/1
  Control C/1 -> Logical Operator5/3, Logical Operator1/3

== system course project/Register9/JCK-Trigger3 ==
  Set J : Inport
  Control C : Inport  Port=2
  Reset K : Inport  Port=3
  Logical Operator1 : Logic  Operator=NAND  Inputs=3  AllPortsSameDT=off  OutDataTypeStr=boolean
  Logical Operator2 : Logic  Operator=NAND  AllPortsSameDT=off  OutDataTypeStr=boolean
  Logical Operator3 : Logic  Operator=NAND  AllPortsSameDT=off  OutDataTypeStr=boolean
  Logical Operator5 : Logic  Operator=NAND  Inputs=3  AllPortsSameDT=off  OutDataTypeStr=boolean
  Memory : Memory
  Non-Inverted : Outport
  wires:
  Memory/1 -> Logical Operator5/2, Logical Operator3/1  "Feedback"
  Logical Operator1/1 -> Logical Operator2/1  "R"
  Logical Operator2/1 -> Non-Inverted/1, Memory/1
  Logical Operator3/1 -> Logical Operator1/2, Logical Operator2/2  "Feedback"
  Logical Operator5/1 -> Logical Operator3/2
  Set J/1 -> Logical Operator1/1
  Reset K/1 -> Logical Operator5/1
  Control C/1 -> Logical Operator5/3, Logical Operator1/3
